simulink model "Lab05Sim"  (R2020b)
settings: Solver=VariableStepAuto  StartTime=0  StopTime=6  MaxStep=0.05  RelTol=1e-3
values from neighbouring files (symbols this model uses):
  a = 1    [Lab05.m]
  b = 1    [Lab05.m]
  du = 1    [Lab05.m]
  ksi = tabksi(i)    [Lab05.m]
  t0 = 0    [Lab05.m]
  ts = 10    [Lab05.m]
  u0 = 0    [Lab05.m]
  w = omega    (= 5)    [Lab05.m]
settings Model: Creator=Lab320  LastModifiedBy=Lab320

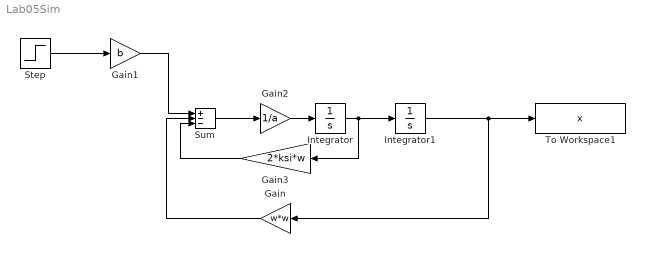
== system Lab05Sim ==
  Gain : Gain  Gain=w*w
  Gain1 : Gain  Gain=b
  Gain2 : Gain  Gain=1/a
  Gain3 : Gain  Gain=2*ksi*w
  Integrator : Integrator
  Integrator1 : Integrator
  Step : Step  Time=t0  Before=u0  After=u0+du  SampleTime=ts
  Sum : Sum  Inputs=+--
  To Workspace1 : ToWorkspace  VariableName=x  SampleTime=-1
  wires:
  Integrator/1 -> Gain3/1, Integrator1/1
  Gain/1 -> Sum/2
  Step/1 -> Gain1/1
  Gain1/1 -> Sum/1
  Sum/1 -> Gain2/1
  Gain2/1 -> Integrator/1
  Integrator1/1 -> To Workspace1/1, Gain/1
  Gain3/1 -> Sum/3
